simulink model "DPCM"  (R2016b)
settings: Solver=VariableStepAuto  StartTime=0.0  StopTime=10.0  RelTol=1e-3
libraries: commsrccod2 x1, dsparch4 x1, commutil2 x1
settings Model: Creator=white  LastModifiedBy=white

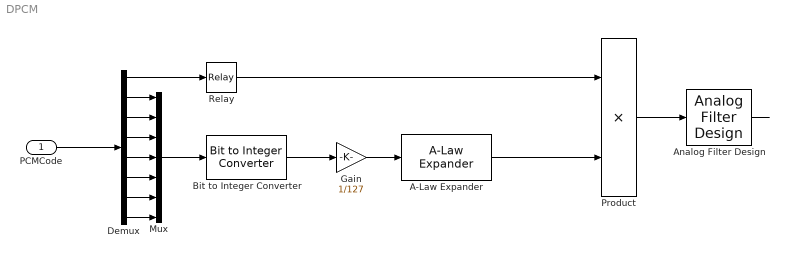
== system DPCM ==
  PCMCode : Inport
  A-Law Expander : commsrccod2/A-Law Expander  A=87.6  V=1
  Analog Filter Design : dsparch4/Analog Filter Design  method=Butterworth  filttype=Lowpass  N=8  Wlo=2*150*pi  Whi=80  Rp=2  Rs=40
  Bit to Integer Converter : commutil2/Bit to Integer Converter  nbits=7  bitOrder=MSB first  signedOutputValues=Unsigned  outDtype=Inherit via internal rule  outDtypeSigned=Inherit via internal rule
  Demux : Demux  Outputs=8
  Gain : Gain  Gain=1/127
  Mux : Mux  Inputs=7
  Product : Product
  Relay : Relay  OnSwitchValue=0.5  OffSwitchValue=0.5  OnOutputValue=-1  OffOutputValue=1
  wires:
  PCMCode/1 -> Demux/1
  Demux/2 -> Mux/1
  Demux/3 -> Mux/2
  Demux/4 -> Mux/3
  Demux/5 -> Mux/4
  Demux/6 -> Mux/5
  Demux/7 -> Mux/6
  Demux/8 -> Mux/7
  Mux/1 -> Bit to Integer Converter/1
  Demux/1 -> Relay/1
  Bit to Integer Converter/1 -> Gain/1
  Gain/1 -> A-Law Expander/1
  Relay/1 -> Product/1
  A-Law Expander/1 -> Product/2
  Product/1 -> Analog Filter Design/1
  Analog Filter Design/1 -> ?
